simulink model "encoder_arduino_test"  (R2023b)
settings: Solver=ode3  StartTime=0.0  StopTime=inf  FixedStep=0.01  RelTol=1e-3  EnableMultiTasking=on
undefined symbols (not defined in the file): K, ref
libraries: arduinolib x3
settings Model: ExtModeTrigDuration=2  Creator=mbelge  LastModifiedBy=Ahmed
settings SolverCC: AlgebraicLoopSolver=TrustRegion
settings DataIOCC: LimitDataPoints=on  SaveFormat=Array  ReturnWorkspaceOutputs=off
settings OptimizationCC: EnhancedBackFolding=on  PassReuseOutputArgsAs=Individual arguments  ZeroExternalMemoryAtStartup=off  ZeroInternalMemoryAtStartup=off  MaxStackSize=64  OptimizeBlockOrder=speed  DifferentSizesBufferReuse=on  OptimizationCustomize=off  EfficientTunableParamExpr=on
settings DebuggingCC: UnderspecifiedInitializationDetection=Classic  MergeDetectMultiDrivingBlocksExec=none  ParameterPrecisionLossMsg=none  ParameterTunabilityLossMsg=error  UnconnectedInputMsg=warning  UnconnectedOutputMsg=warning  UnconnectedLineMsg=warning  SFUnexpectedBacktrackingDiag=warning  SFNoUnconditionalDefaultTransitionDiag=warning  SFExecutionAtInitializationDiag=none  ArithmeticOperatorsInVariantConditions=warning
settings HardwareCC: ProdBitPerInt=16  ProdBitPerPointer=16  ProdBitPerSizeT=16  ProdBitPerPtrDiffT=16  ProdLargestAtomicFloat=None  ProdWordSize=8  ProdHWDeviceType=Atmel->AVR
settings ModelReferenceCC: PropagateSignalLabelsOutOfModel=off
settings SFSimCC: SimUseLocalCustomCode=off  MATLABDynamicMemAlloc=off  CustomCodeUndefinedFunction=UseInterfaceOnly
settings RTWCC: Description=Embedded Coder  SystemTargetFile=ert.tlc  HardwareBoard=Arduino Mega 2560  TemplateMakefile=ert_default_tmf  RTWVerbose=off  RTWUseLocalCustomCode=off  Toolchain=Arduino AVR  BuildConfiguration=Faster Runs
settings CodeAppCC: ForceParamTrailComments=on  IgnoreCustomStorageClasses=off  OperatorAnnotations=on  SimulinkDataObjDesc=on  SFDataObjDesc=on  InsertBlockDesc=on
settings ERTTargetCC: SupportContinuousTime=on  SupportVariableSizeSignals=on  ExtModeTransport=3  ExtModeStaticAlloc=on  ExtModeAutomaticAllocSize=off  ExtModeStaticAllocSize=2048  ExtModeMexFile=ext_xcp  ExtModeIntrfLevel=Level2 - Open
settings ConfigComp: CovMetricSettings=dw  CovSaveCumulativeToWorkspaceVar=on  CovSaveSingleToWorkspaceVar=on  CovExternalEMLEnable=off  CovSFcnEnable=off

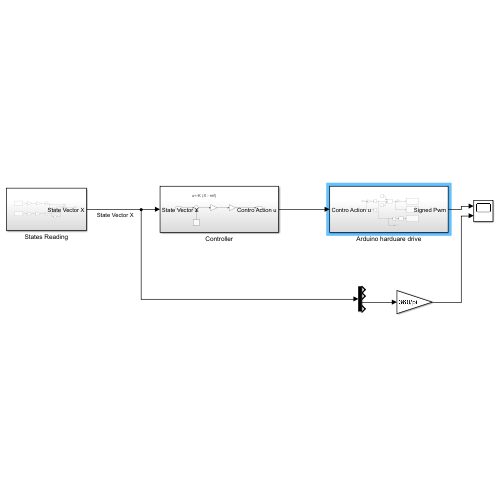
[thumbnail: Simulink's stored preview of the top-level diagram]
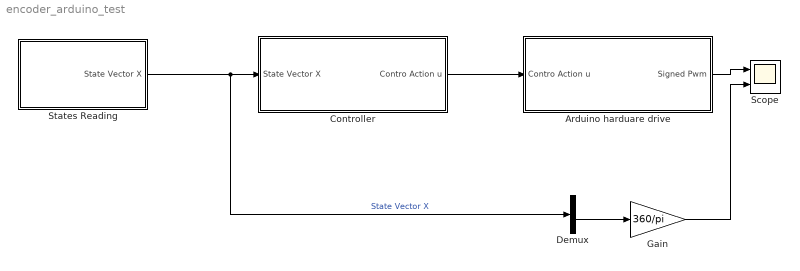
== system encoder_arduino_test ==
  Arduino harduare drive : Subsystem
  Controller : Subsystem
  Demux : Demux
  Gain : Gain  Gain=360/pi
  Scope : Scope  NumInputPorts=2
  States Reading : Subsystem
  wires:
  States Reading/1(State Vector X) -> Demux/1, Controller/1(State Vector X)  "State Vector X"
  Controller/1(Contro Action u) -> Arduino harduare drive/1(Contro Action u)
  Arduino harduare drive/1(Signed Pwm) -> Scope/1
  Demux/3 -> Gain/1
  Gain/1 -> Scope/2

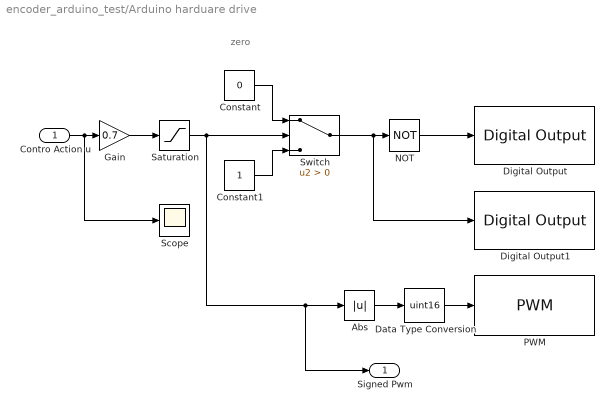
== system encoder_arduino_test/Arduino harduare drive ==
  note: zero
  Contro Action u : Inport
  Abs : Abs  SaturateOnIntegerOverflow=off
  Constant : Constant  Value=0
  Constant1 : Constant
  Data Type Conversion : DataTypeConversion  OutDataTypeStr=uint16  SaturateOnIntegerOverflow=off  RndMeth=Floor
  Digital Output : arduinolib/Digital Output  pinNumber=8  Direction=output  blockPlatform=arduino
  Digital Output1 : arduinolib/Digital Output  pinNumber=7  Direction=output  blockPlatform=arduino
  Gain : Gain  Gain=0.7
  NOT : Logic  Operator=NOT  IconShape=distinctive  AllPortsSameDT=off  OutDataTypeStr=boolean
  PWM : arduinolib/PWM  pinNumber=6  frequencyType=Default  desiredFrequency=490.2  achievableFrequency=490.2
  Saturation : Saturate  UpperLimit=255  LowerLimit=-255
      settings: LockScale=on
  Scope : Scope
  Switch : Switch  Criteria=u2 > Threshold  SaturateOnIntegerOverflow=off  InputSameDT=off
  Signed Pwm : Outport
  wires:
  Contro Action u/1 -> Scope/1, Gain/1
  Saturation/1 -> Signed Pwm/1, Abs/1, Switch/2
  Constant/1 -> Switch/1
  Constant1/1 -> Switch/3
  NOT/1 -> Digital Output/1
  Switch/1 -> Digital Output1/1, NOT/1
  Abs/1 -> Data Type Conversion/1
  Gain/1 -> Saturation/1
  Data Type Conversion/1 -> PWM/1

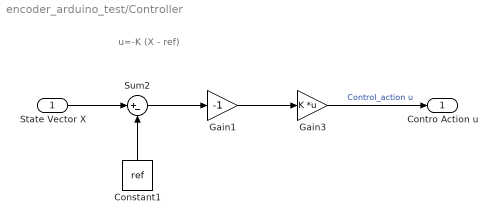
== system encoder_arduino_test/Controller ==
  note: u=-K (X - ref)
  State Vector X : Inport
  Constant1 : Constant  Value=ref
  Gain1 : Gain  Gain=-1
  Gain3 : Gain  Gain=K  Multiplication=Matrix(K*u)
  Sum2 : Sum  Inputs=|+-
  Contro Action u : Outport
  wires:
  Constant1/1 -> Sum2/2
  Sum2/1 -> Gain1/1
  State Vector X/1 -> Sum2/1
  Gain3/1 -> Contro Action u/1  "Control_action u"
  Gain1/1 -> Gain3/1

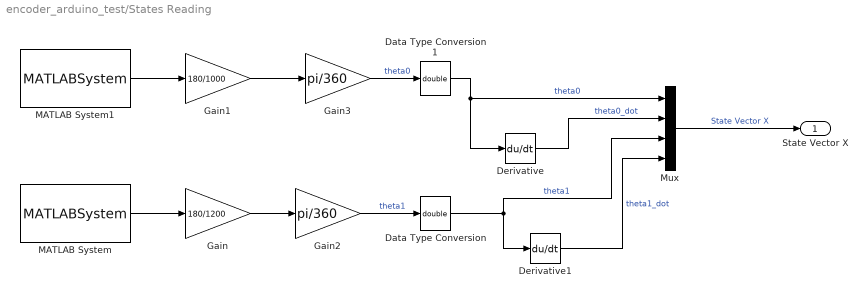
== system encoder_arduino_test/States Reading ==
  Data Type Conversion : DataTypeConversion  OutDataTypeStr=double  SaturateOnIntegerOverflow=off  RndMeth=Floor
  Data Type Conversion1 : DataTypeConversion  OutDataTypeStr=double  SaturateOnIntegerOverflow=off  RndMeth=Floor
  Derivative : Derivative
  Derivative1 : Derivative
  Gain : Gain  Gain=180/1200
  Gain1 : Gain  Gain=180/1000
  Gain2 : Gain  Gain=pi/360
  Gain3 : Gain  Gain=pi/360
  MATLAB System : MATLABSystem  System=Encoder_arduino  Encoder=0  PinA=2  PinB=3  SampleTime=0.01
      mask Type: Encoder_arduino
      mask Display:
      | disp('Encoder');
      | port_label('output',1,'y');
  MATLAB System1 : MATLABSystem  System=Encoder_arduino  Encoder=1  PinA=18  PinB=19  SampleTime=0.01
      mask Type: Encoder_arduino
      mask Display:
      | disp('Encoder');
      | port_label('output',1,'y');
  Mux : Mux
  State Vector X : Outport
  wires:
  MATLAB System1/1 -> Gain1/1
  Data Type Conversion1/1 -> Derivative/1, Mux/1  "theta0"
  Gain/1 -> Gain2/1
  Derivative/1 -> Mux/2  "theta0_dot"
  MATLAB System/1 -> Gain/1
  Derivative1/1 -> Mux/4  "theta1_dot"
  Data Type Conversion/1 -> Derivative1/1, Mux/3  "theta1"
  Gain1/1 -> Gain3/1
  Gain2/1 -> Data Type Conversion/1  "theta1"
  Gain3/1 -> Data Type Conversion1/1  "theta0"
  Mux/1 -> State Vector X/1  "State Vector X"
